simulink model "PM_fnc18_DevHarness_Xload_1Dlookup"  (R2022a)
settings: Solver=FixedStepAuto  StartTime=0.0  StopTime=inf  FixedStep=0.05  RelTol=1e-3
model workspace (MAT data in the model file):
  table_Xload_dur_ms = Simulink.LookupTable
  table_Xload_dur_ms.Table = Simulink.lookuptable.Table
  table_Xload_dur_ms.Table.Value = [8820; 4050; 3000; 2430; 2010; 1000; 500; 200; 100; 50; 10]
  table_Xload_dur_ms.Table.Dimensions = [11 1]
  table_Xload_dur_ms.Table.DataType = 'uint16'
  table_Xload_dur_ms.Table.Min = 0
  table_Xload_dur_ms.Table.Max = 8820
  table_Xload_dur_ms.Table.Unit = 'msec'
  table_Xload_dur_ms.Table.FieldName = 'cal_table_vals_Xload_dur_ms'
  table_Xload_dur_ms.Breakpoints = Simulink.lookuptable.Breakpoint
  table_Xload_dur_ms.Breakpoints.Value = [105; 155; 180; 200; 220; 440; 880; 1100; 1300; 1500; 1700]
  table_Xload_dur_ms.Breakpoints.TunableSizeName = 'N1'
  table_Xload_dur_ms.Breakpoints.Dimensions = [11 1]
  table_Xload_dur_ms.Breakpoints.DataType = 'int16'
  table_Xload_dur_ms.Breakpoints.Min = 0
  table_Xload_dur_ms.Breakpoints.Max = 1700
  table_Xload_dur_ms.Breakpoints.Unit = 'A'
  table_Xload_dur_ms.Breakpoints.FieldName = 'cal_table_bkpts_Xload_amps_A'
  table_Xload_dur_ms.SupportTunableSize = 0
  table_Xload_dur_ms.StructTypeInfo = Simulink.lookuptable.StructTypeInfo
  table_Xload_dur_ms.StructTypeInfo.Name = 'Xload_dur_ms'
  table_Xload_dur_ms.StructTypeInfo.DataScope = 'Auto'
libraries: PM_lib x1
settings Model: PacingRate=1.600000  Creator=306427  LastModifiedBy=306427

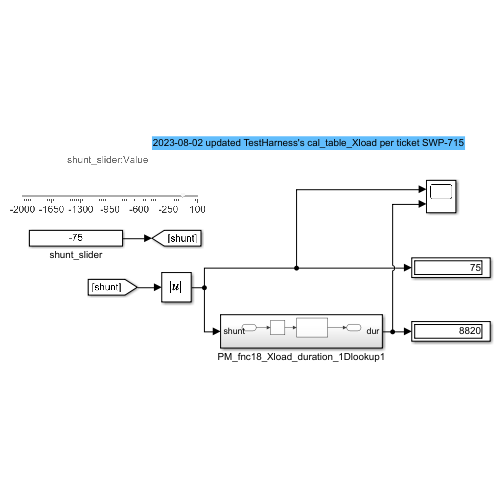
[thumbnail: Simulink's stored preview of the top-level diagram]
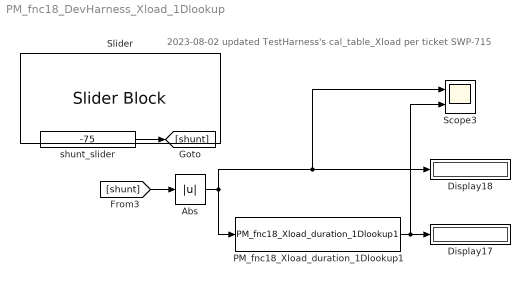
== system PM_fnc18_DevHarness_Xload_1Dlookup ==
  note: 2023-08-02 updated TestHarness's cal_table_Xload per ticket SWP-715
  Abs : Abs  SaturateOnIntegerOverflow=off
  Display17 : Display
  Display18 : Display
  PM_fnc18_Xload_duration_1Dlookup1 : PM_lib/PM_fnc18_Xload_duration_1Dlookup1  SystemSampleTime=-1  VariantActivationTime=update diagram  Latency=0  AutoFrameSizeCalculation=off
      link override cal_table_Xload: OutMax=8820
  Scope3 : Scope  NumInputPorts=2
  Slider : SliderBlock  ScaleMin=-2000
  shunt_slider : Constant  Value=-75
  wires:
  PM_fnc18_Xload_duration_1Dlookup1/1 -> Scope3/2, Display17/1
  Abs/1 -> PM_fnc18_Xload_duration_1Dlookup1/1, Scope3/1, Display18/1
  [shunt] -> Abs/1
  shunt_slider/1 -> [shunt]
